simulink model "trajectory_test_v_1"  (R2016a)
settings: Solver=FixedStepDiscrete  StartTime=0.0  StopTime=inf  FixedStep=0.001  RelTol=1e-3
InitFcn:
  | cd(fileparts(which(bdroot)));
  | 
  | init_model
StartFcn:
  | cd(fileparts(which(bdroot)));
model workspace (MAT data in the model file):
  par.dimensions.torso_width = 0.111490833
  par.dimensions.pelvis_width = 0.135213424
  par.dimensions.pelvis_depth = 0.207340833
  par.dimensions.upper_length = 0.4
  par.dimensions.lower_length = 0.535
  par.dimensions.foot_height = 0.05
  par.dimensions.leg_length = 0.934
  par.encoder_limit.RHAA.abduction = 180694
  par.encoder_limit.RHAA.adduction = 63590
  par.encoder_limit.RHFE.flexion = 437000
  par.encoder_limit.RHFE.extension = 61029
  par.encoder_limit.RKFE.flexion = 59910
  par.encoder_limit.RKFE.extension = 415850
  par.encoder_limit.LHAA.abduction = 729800
  par.encoder_limit.LHAA.adduction = 847900
  par.encoder_limit.LHFE.flexion = 344400
  par.encoder_limit.LHFE.extension = 718630
  par.encoder_limit.LKFE.flexion = 720100
  par.encoder_limit.LKFE.extension = 365270
  par.jointAngle_limit.RHAA.abduction = 0.331612557879
  par.jointAngle_limit.RHAA.adduction = -0.383972435439
  par.jointAngle_limit.RHFE.flexion = 0.575958653158
  par.jointAngle_limit.RHFE.extension = -2.11184839491
  par.jointAngle_limit.RKFE.flexion = -0.0261799387799
  par.jointAngle_limit.RKFE.extension = 2.32128790515
  par.jointAngle_limit.LHAA.abduction = 0.331612557879
  par.jointAngle_limit.LHAA.adduction = -0.383972435439
  par.jointAngle_limit.LHFE.flexion = 0.575958653158
  par.jointAngle_limit.LHFE.extension = -2.11184839491
  par.jointAngle_limit.LKFE.flexion = -0.0261799387799
  par.jointAngle_limit.LKFE.extension = 2.32128790515
  par.joint_limit_min = [-0.349065850399 -1.90240888467 -0.0523598775598 -0.401425727959 -1.90240888467 -0.0523598775598]
  par.joint_limit_max = [0.401425727959 0.366519142919 2.11184839491 0.349065850399 0.366519142919 2.11184839491]
  tol = 0.001
undefined symbols (not defined in the file or in its folder): Right_Leg
libraries: xpcethercatlib x11, slrtlib x3, aerolibanimutils x1
settings Model: xpc_rtwmakecfg_data=_xpcethercatlib_  SimulationMode=external  Creator=Projectmarch  LastModifiedBy=Projectmarch
settings SolverCC: EnableConcurrentExecution=on
settings DataIOCC: SaveFormat=StructureWithTime
settings OptimizationCC: BlockReduction=off  OptimizeBlockIOStorage=off  BufferReuse=off  GlobalBufferReuse=off  ExpressionFolding=off  LocalBlockOutputs=off
settings HardwareCC: ProdBitPerPointer=32  ProdLargestAtomicFloat=None  ProdWordSize=32  ProdLongLongMode=on  ProdHWDeviceType=Generic->32-bit x86 compatible
settings RTWCC: SystemTargetFile=slrt.tlc  TemplateMakefile=slrt_default_tmf  Description=Simulink Real-Time

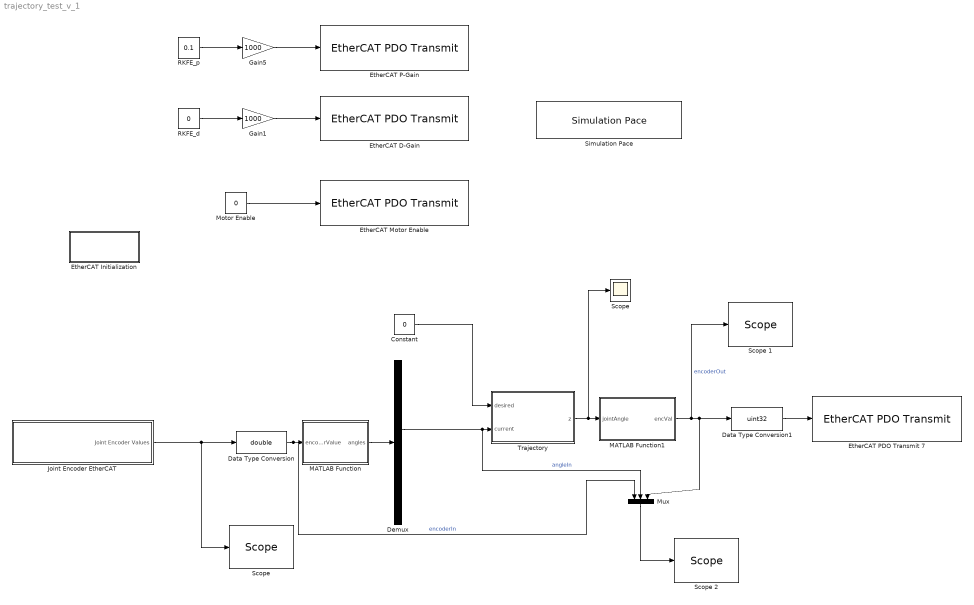
== system trajectory_test_v_1 ==
  Constant : Constant  Value=0
  Data Type Conversion : DataTypeConversion  OutDataTypeStr=double
  Data Type Conversion1 : DataTypeConversion  OutDataTypeStr=uint32
  Demux : Demux  Outputs=6
  EtherCAT D-Gain : xpcethercatlib/EtherCAT PDO Transmit   Priority=3  sig_name=Right_Leg.Outputs.K_data[3]  sig_offset=2344  sig_type=int32  type_size=32  sig_dim=1  device_id=0  sample_time=0.001000
  EtherCAT Initialization : Subsystem
  EtherCAT Motor Enable : xpcethercatlib/EtherCAT PDO Transmit   Priority=3  sig_name=Right_Leg.Outputs.K_motorEnable  sig_offset=2168  sig_type=uint8  type_size=8  sig_dim=1  device_id=0  sample_time=0.001000
  EtherCAT P-Gain : xpcethercatlib/EtherCAT PDO Transmit   Priority=3  sig_name=Right_Leg.Outputs.K_data[1]  sig_offset=2280  sig_type=int32  type_size=32  sig_dim=1  device_id=0  sample_time=0.001000
  EtherCAT PDO Transmit 7 : xpcethercatlib/EtherCAT PDO Transmit   Priority=3  sig_name=Right_Leg.Outputs.K_jointSetPoint  sig_offset=2136  sig_type=uint32  type_size=32  sig_dim=1  device_id=0  sample_time=0.001000
  Gain1 : Gain  Gain=1000  OutDataTypeStr=int32
  Gain5 : Gain  Gain=1000  OutDataTypeStr=int32
  Joint Encoder EtherCAT : Subsystem
  MATLAB Function : MATLAB Function  TreatAsAtomicUnit=on
  MATLAB Function1 : MATLAB Function  TreatAsAtomicUnit=on
  Motor Enable : Constant  Value=0  OutDataTypeStr=Inherit: Inherit via back propagation
  Mux : Mux  Inputs=3
  RKFE_d : Constant  Value=0  OutDataTypeStr=int32
  RKFE_p : Constant  Value=0.1  OutDataTypeStr=int32
  Scope : Scope
  "Scope " : slrtlib/Displays and Logging/Scope   scopeno=1  scopetype=Target  autostart=on  viewmode=Graphical sliding  formatstr='%15.6f'  grid=on  ylimits=[0,0]  nosamples=25000  noprepostsamples=0  interleave=1  triggermode=FreeRun  triggersignal=1  trigsignalfromport=off  triggerlevel=0.0  triggerslope=Either  triggerscope=1  triggersample=0  filename=data.dat  mode=Lazy  writesize=512  autorestart=off  dynamicfilemode=off  maxwritefilesize=512*1024^2
  Scope 1 : slrtlib/Displays and Logging/Scope   scopeno=2  scopetype=Target  autostart=on  viewmode=Graphical sliding  formatstr='%15.6f'  grid=on  ylimits=[0,0]  nosamples=25000  noprepostsamples=0  interleave=1  triggermode=FreeRun  triggersignal=1  trigsignalfromport=off  triggerlevel=0.0  triggerslope=Either  triggerscope=1  triggersample=0  filename=data.dat  mode=Lazy  writesize=512  autorestart=off  dynamicfilemode=off  maxwritefilesize=512*1024^2
  Scope 2 : slrtlib/Displays and Logging/Scope   scopeno=3  scopetype=Target  autostart=on  viewmode=Numerical  formatstr='%15.6f'  grid=on  ylimits=[0,0]  nosamples=250  noprepostsamples=0  interleave=1  triggermode=FreeRun  triggersignal=1  trigsignalfromport=off  triggerlevel=0.0  triggerslope=Either  triggerscope=1  triggersample=0  filename=data.dat  mode=Lazy  writesize=512  autorestart=off  dynamicfilemode=off  maxwritefilesize=512*1024^2
  Simulation Pace : aerolibanimutils/Simulation Pace  SimulationPace=1  SleepMode=MATLAB Thread  OutputPaceError=off  SampleTime=-1
  Trajectory : MATLAB Function  TreatAsAtomicUnit=on
  wires:
  RKFE_p/1 -> Gain5/1
  Gain5/1 -> EtherCAT P-Gain/1
  Joint Encoder EtherCAT/1(Joint Encoder Values) -> "Scope "/1, Data Type Conversion/1
  MATLAB Function/1(angles) -> Demux/1
  Data Type Conversion/1 -> Mux/1, MATLAB Function/1(encoderValue)  "encoderIn"
  Constant/1 -> Trajectory/1(desired)
  Trajectory/1(z) -> Scope/1, MATLAB Function1/1(jointAngle)
  MATLAB Function1/1(encVal) -> Scope 1/1, Mux/3, Data Type Conversion1/1  "encoderOut"
  Data Type Conversion1/1 -> EtherCAT PDO Transmit 7/1
  RKFE_d/1 -> Gain1/1
  Gain1/1 -> EtherCAT D-Gain/1
  Demux/3 -> Mux/2, Trajectory/2(current)  "angleIn"
  Motor Enable/1 -> EtherCAT Motor Enable/1
  Mux/1 -> Scope 2/1

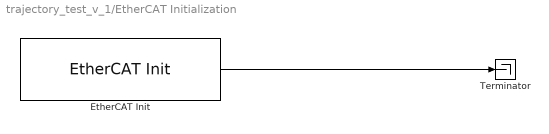
== system trajectory_test_v_1/EtherCAT Initialization ==
  EtherCAT Init : xpcethercatlib/EtherCAT Init   Priority=0  config_file=D:\Software\MATLAB\simulink-models\EtherCAT Config files\full_setup_v1.0.xml  device_id=0  pci_bus=2  pci_slot=0  dctuning=0  enaDebug=off  enaDC=on  errLink=on  masterDbg=on  stateChgDbg=on  baseClock=off  masterCfg=off  logFile='c:\dbglog.txt'  sample_time=0.001000
  Terminator : Terminator
  wires:
  EtherCAT Init/1 -> Terminator/1

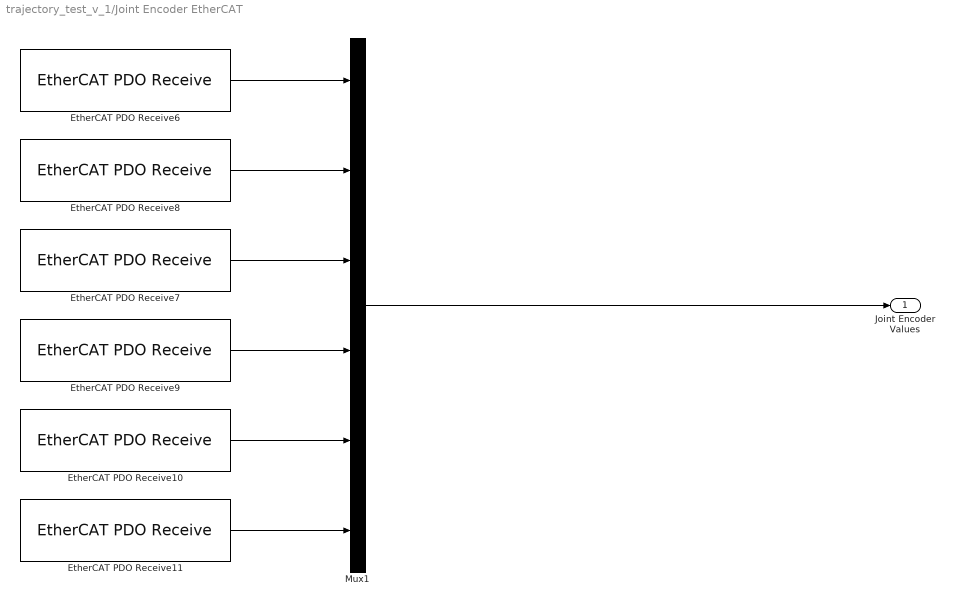
== system trajectory_test_v_1/Joint Encoder EtherCAT ==
  EtherCAT PDO Receive10 : xpcethercatlib/EtherCAT PDO Receive  Priority=2  sig_name=Left_Leg.Inputs.H_jointAngle  sig_offset=1144  sig_type=uint32  type_size=32  sig_dim=1  device_id=0  sample_time=0.001000
  EtherCAT PDO Receive11 : xpcethercatlib/EtherCAT PDO Receive  Priority=2  sig_name=Left_Leg.Inputs.K_jointAngle  sig_offset=1312  sig_type=uint32  type_size=32  sig_dim=1  device_id=0  sample_time=0.001000
  EtherCAT PDO Receive6 : xpcethercatlib/EtherCAT PDO Receive  Priority=2  sig_name=Hip_HAA.Inputs.R_jointAngle  sig_offset=688  sig_type=uint32  type_size=32  sig_dim=1  device_id=0  sample_time=0.001000
  EtherCAT PDO Receive7 : xpcethercatlib/EtherCAT PDO Receive  Priority=2  sig_name=Right_Leg.Inputs.K_jointAngle  sig_offset=2000  sig_type=uint32  type_size=32  sig_dim=1  device_id=0  sample_time=0.001000
  EtherCAT PDO Receive8 : xpcethercatlib/EtherCAT PDO Receive  Priority=2  sig_name=Right_Leg.Inputs.H_jointAngle  sig_offset=1832  sig_type=uint32  type_size=32  sig_dim=1  device_id=0  sample_time=0.001000
  EtherCAT PDO Receive9 : xpcethercatlib/EtherCAT PDO Receive  Priority=2  sig_name=Hip_HAA.Inputs.L_jointAngle  sig_offset=208  sig_type=uint32  type_size=32  sig_dim=1  device_id=0  sample_time=0.001000
  Mux1 : Mux  Inputs=6
  Joint Encoder Values : Outport
  wires:
  EtherCAT PDO Receive7/1 -> Mux1/3
  EtherCAT PDO Receive9/1 -> Mux1/4
  EtherCAT PDO Receive8/1 -> Mux1/2
  EtherCAT PDO Receive6/1 -> Mux1/1
  EtherCAT PDO Receive10/1 -> Mux1/5
  EtherCAT PDO Receive11/1 -> Mux1/6
  Mux1/1 -> Joint Encoder Values/1

== matlab function trajectory_test_v_1/Trajectory ==
  data: desired input; current input; z output
function z = fcn(desired, current)
%#codegen
persistent i setpoint flag trajectory

samples = 3000;

if (isempty(i))
    i = 0;
    flag = -1;
    setpoint = desired;
    trajectory = linspace(current, current, samples);
end

if(setpoint ~= desired)
    trajectory = linspace(current, desired, samples);
    setpoint = desired;
    i = 0;
end


if i < length(trajectory)
   i = i+1;
end

z = trajectory(i); 
if( z == 0)
    z = current;
end

== matlab function trajectory_test_v_1/MATLAB Function ==
  data: encoderValue input; angles output; par parameter
function angles = convertToJointAngles(encoderValue, par)
angles = zeros(6,1);

for i = 1:6
    angles(i) = enc2rad(encoderValue(i), i, par);
end

== matlab function trajectory_test_v_1/MATLAB Function1 ==
  data: jointAngle input; encVal output; par parameter
function encVal = convertToEncoderValues(jointAngle, par)

encVal = rad2enc(jointAngle, 3, par);
